simulink model "elasticband"  (Simulink 9.2)
settings: Solver=ode45  StartTime=0.0  StopTime=60  MaxStep=1e-2  RelTol=1e-6
settings Model: Creator=jinwooro  LastModifiedBy=jinwooro  PauseTimes=28  NumberOfSteps=5
settings DataIOCC: LimitDataPoints=off  SaveFormat=Dataset  SignalLoggingSaveFormat=Dataset
settings OptimizationCC: LifeSpan=auto
settings DebuggingCC: UnderspecifiedInitializationDetection=Simplified  MergeDetectMultiDrivingBlocksExec=error  FcnCallInpInsideContextMsg=error  StateNameClashWarn=none  SFUnexpectedBacktrackingDiag=error  SFNoUnconditionalDefaultTransitionDiag=error  SFExecutionAtInitializationDiag=warning
settings HardwareCC: ProdBitPerPointer=64  ProdBitPerSizeT=64  ProdBitPerPtrDiffT=64  ProdLargestAtomicFloat=Float  ProdIntDivRoundTo=Zero  ProdEndianess=LittleEndian  ProdWordSize=64  ProdHWDeviceType=Intel->x86-64 (Windows64)
settings ModelReferenceCC: PropagateSignalLabelsOutOfModel=on
settings SFSimCC: SimUseLocalCustomCode=on
settings RTWCC: RTWUseLocalCustomCode=on
settings CodeAppCC: StateflowObjectComments=off
settings GRTTargetCC: TargetLangStandard=C99 (ISO)  GeneratePreprocessorConditionals=Use local settings  CombineOutputUpdateFcns=on  GRTInterface=off
settings ConfigComp: CovMetricSettings=dwe  CovHtmlReporting=off  CovSaveCumulativeToWorkspaceVar=off  CovSaveSingleToWorkspaceVar=off  CovExternalEMLEnable=on

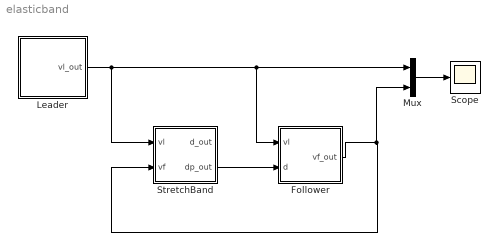
== system elasticband ==
  Follower : Stateflow chart  TreatAsAtomicUnit=on
  Leader : Stateflow chart  TreatAsAtomicUnit=on
  Mux : Mux  Inputs=2
  Scope : Scope
  StretchBand : Stateflow chart  TreatAsAtomicUnit=on
  wires:
  Leader/1(vl_out) -> Follower/1(vl), Mux/1, StretchBand/1(vl)
  Mux/1 -> Scope/1
  StretchBand/2(dp_out) -> Follower/2(d)
  Follower/1(vf_out) -> StretchBand/2(vf), Mux/2

== stateflow chart Follower ==
  settings: updateMethod=CONTINUOUS
  state ACC
    du:
    vf_dot = 0.7 * (d - 10) + (vl - vf) * 0.7;
    vf_out = vf;
  state Stop
    du:
    vf_dot = 0;
    vf_out = vf;
  state Emergency
    du:
    vf_dot = -6;
    vf_out = vf;
  (default) -> ACC : {vf = 17;}
  Stop -> ACC : [d > 15]{vf = 0.001;}
  ACC -> Stop [order 2] : [vf <= 0]{vf = 0;}
  ACC -> Emergency [order 1] : [ power(2 * (d - 2) / 6, 0.5) <= 1]
  Emergency -> Stop : [ vf <= 0 ]
  data: vl input double; vf local double; vf_out output double; d input double
  data vf settings: updateMethod=SF_CONTINUOUS_TIME_DATA

== stateflow chart StretchBand ==
  settings: updateMethod=CONTINUOUS
  state OverEstimate
    du:
    d_dot = vl - vf;
    d_out = d;
    dp_out = d * 1.05;
  state Normal
    du:
    d_dot = vl - vf;
    d_out = d;
    dp_out = d;
  (default) -> OverEstimate : {d = 20;}
  OverEstimate -> Normal : [d <= 10]
  Normal -> OverEstimate : [d > 10]
  data: d local double; d_out output double; vl input double; vf input double; dp_out output double
  data d settings: updateMethod=SF_CONTINUOUS_TIME_DATA

== stateflow chart Leader ==
  settings: updateMethod=CONTINUOUS
  state ConstAcc
    du:
    vl_dot = -3 * cos(3 * pi * tau) + 3;
    tau_dot = 0;
    vl_out = vl;
  state IncAcc
    du:
    vl_dot = -3 * cos(3 * pi * tau) + 3;
    tau_dot = 1;
    vl_out = vl;
  state DecAcc
    du:
    vl_dot = - 0.7 * vl * (1 - vl / 17) - 0.2;
    tau_dot = 0;
    vl_out = vl;
  IncAcc -> ConstAcc : [-cos(3 * pi * tau) >= 0.99]
  ConstAcc -> DecAcc : [vl >= 17]
  (default) -> DecAcc : {vl = 17;
      | tau = 0;}
  DecAcc -> IncAcc : [vl <= 0 ]{tau = 0;}
  data: vl local double; vl_out output double; tau local double
  data vl settings: updateMethod=SF_CONTINUOUS_TIME_DATA
  data tau settings: updateMethod=SF_CONTINUOUS_TIME_DATA
